simulink model "BLDC_motor"  (R2015b)
settings: Solver=VariableStepAuto  StartTime=0.0  StopTime=0.2  RelTol=1e-3
libraries: powerlib x15
settings Model: Creator=Meghdeep  LastModifiedBy=Jana

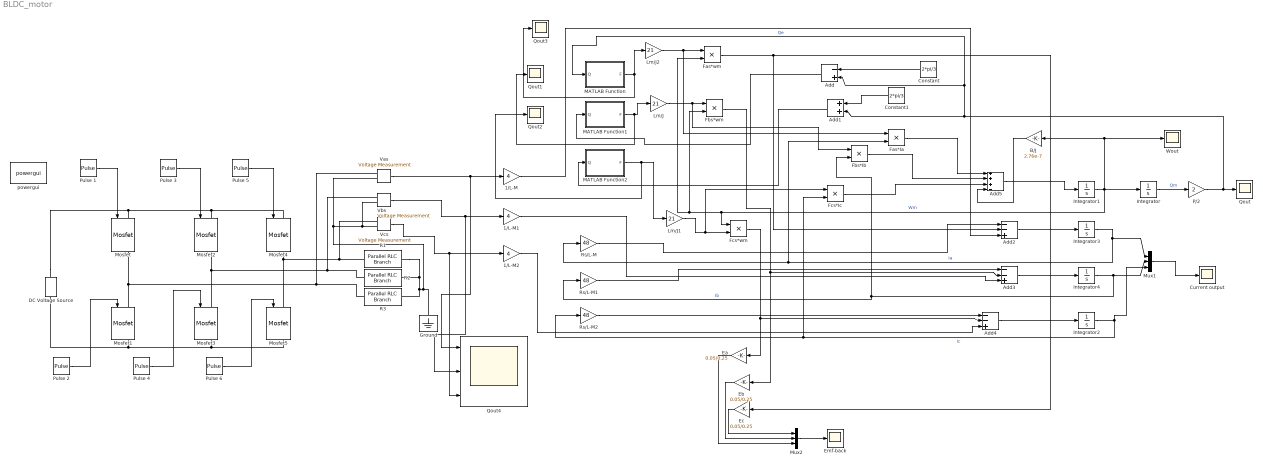
== system BLDC_motor ==
  1/L-M : Gain  Gain=4
  1/L-M1 : Gain  Gain=4
  1/L-M2 : Gain  Gain=4
  Add : Sum  Inputs=-+
  Add1 : Sum
  Add2 : Sum  Inputs=--+
  Add3 : Sum  Inputs=--+
  Add4 : Sum  Inputs=--+
  Add5 : Sum  Inputs=+++-
  B/J : Gain  Gain=2.76e-7
  Constant : Constant  Value=2*pi/3
  Constant1 : Constant  Value=2*pi/3
  Current output : Scope
  DC Voltage Source : powerlib/Electrical Sources/DC Voltage Source  Amplitude=10  Measurements=None
  Ea : Gain  Gain=0.05/0.25
  Eb : Gain  Gain=0.05/0.25
  Ec : Gain  Gain=0.05/0.25
  Emf-back : Scope
  Fas*Ia : Product
  Fas*wm : Product
  Fbs*Ib : Product
  Fbs*wm : Product
  Fcs*Ic : Product
  Fcs*wm : Product
  Ground : powerlib/Elements/Ground  LConnTagsString=a
  Integrator{,1..4} (5 alike) : Integrator
  Lm/J : Gain  Gain=21
  Lm/J1 : Gain  Gain=21
  Lm/J2 : Gain  Gain=21
  MATLAB Function : MATLAB Function  TreatAsAtomicUnit=on
  MATLAB Function1 : MATLAB Function  TreatAsAtomicUnit=on
  MATLAB Function2 : MATLAB Function  TreatAsAtomicUnit=on
  Mosfet{,1..5} (6 alike) : powerlib/Power Electronics/Mosfet  Ron=0.1  Lon=0  Rd=0.01  Vfd=0  IC=0  Rs=1e5  Cs=inf  Measurements=on
  Mux1 : Mux  Inputs=3
  Mux2 : Mux  Inputs=3
  P/2 : Gain  Gain=2
  Pulse 1 : DiscretePulseGenerator  PulseType=Time based  Amplitude=10  Period=0.02  PulseWidth=100/3
  Pulse 2 : DiscretePulseGenerator  PulseType=Time based  Amplitude=10  Period=0.02  PulseWidth=100/3  PhaseDelay=0.0033
  Pulse 3 : DiscretePulseGenerator  PulseType=Time based  Amplitude=10  Period=0.02  PulseWidth=100/3  PhaseDelay=0.0067
  Pulse 4 : DiscretePulseGenerator  PulseType=Time based  Amplitude=10  Period=0.02  PulseWidth=100/3  PhaseDelay=0.01
  Pulse 5 : DiscretePulseGenerator  PulseType=Time based  Amplitude=10  Period=0.02  PulseWidth=100/3  PhaseDelay=0.0133
  Pulse 6 : DiscretePulseGenerator  PulseType=Time based  Amplitude=10  Period=0.02  PulseWidth=100/3  PhaseDelay=0.0167
  Qout{,1..3} (4 alike) : Scope
  Qout4 : Scope  NumInputPorts=3
  R1 : powerlib/Elements/Parallel RLC Branch  LConnTagsString=a  RConnTagsString=__new0  BranchType=R  Resistance=1  Inductance=1e-3  SetiL0=off  InitialCurrent=0  Capacitance=1e-6  Setx0=off  InitialVoltage=0  Measurements=None
  R2 : powerlib/Elements/Parallel RLC Branch  LConnTagsString=a  RConnTagsString=__new0  BranchType=R  Resistance=1  Inductance=1e-3  SetiL0=off  InitialCurrent=0  Capacitance=1e-6  Setx0=off  InitialVoltage=0  Measurements=None
  R3 : powerlib/Elements/Parallel RLC Branch  LConnTagsString=a  RConnTagsString=__new0  BranchType=R  Resistance=1  Inductance=1e-3  SetiL0=off  InitialCurrent=0  Capacitance=1e-6  Setx0=off  InitialVoltage=0  Measurements=None
  Rs/L-M : Gain  Gain=48
  Rs/L-M1 : Gain  Gain=48
  Rs/L-M2 : Gain  Gain=48
  Vas : powerlib/Measurements/Voltage Measurement  PhasorSimulation=off  OutputType=Complex  PSBequivalent=0
  Vbs : powerlib/Measurements/Voltage Measurement  PhasorSimulation=off  OutputType=Complex  PSBequivalent=0
  Vcs : powerlib/Measurements/Voltage Measurement  PhasorSimulation=off  OutputType=Complex  PSBequivalent=0
  Wout : Scope
  powergui : powerlib/powergui  Priority=1  SimulationMode=Continuous  SolverType=Tustin/Backward Euler (TBE)  SampleTime=50e-6  frequency=60  SPID=off  DisableSnubberDevices=off  DisableRonSwitches=off  DisableVfSwitches=off  SwTol=0  DisplayEquations=off  Interpol=off  ExternalGateDelay=off  methode=off  Ts=10  FunctionMessages=off  echomessages=off  HookPort=off  EnableUseOfTLC=off  x0status=blocks  frequencyindice=0  Pbase=100e6  ErrMax=1e-4  Iterations=50  UnitsV=kV  UnitsW=MW  buscounter=0  RestoreLinks=warning  ResistiveCurrentMeasurement=off  Frange=[0:2:500]  Ylog=off  Xlog=on  ShowGrid=off  save=off  variable=ZData  structure=0  ZoomFFT=off  StartTime=0.0  cycles=1  DisplayStyle=1  fundamental=60  FreqAxis=off  MaxFrequency=1000  frequencyindicesteady=1  RmsSteady=1  display=off
  wires:
  Integrator1/1 -> B/J/1, Wout/1, Integrator/1, Fcs*wm/1, Fas*wm/2, Fbs*wm/2  "Wm"
  Integrator3/1 -> Mux1/1, Fas*Ia/2, Rs/L-M/1  "Ia"
  Integrator4/1 -> Mux1/2, Fbs*Ib/2, Rs/L-M1/1  "Ib"
  Integrator2/1 -> Mux1/3, Fcs*Ic/2, Rs/L-M2/1  "Ic"
  Fbs*wm/1 -> Add3/2, Eb/1
  P/2/1 -> Qout/1, MATLAB Function/1(Q), Add/2, Add1/2  "Qe"
  Constant/1 -> Add/1
  Constant1/1 -> Add1/1
  Add/1 -> MATLAB Function1/1(Q)
  Add1/1 -> MATLAB Function2/1(Q)
  Fcs*wm/1 -> Add4/2, Ea/1
  Fas*wm/1 -> Add2/2, Ec/1
  Lm/J2/1 -> Fas*wm/1, Fas*Ia/1
  1/L-M/1 -> Add2/3
  Rs/L-M/1 -> Add2/1
  Add2/1 -> Integrator3/1
  Rs/L-M1/1 -> Add3/1
  Lm/J/1 -> Fbs*Ib/1, Fbs*wm/1
  1/L-M1/1 -> Add3/3
  Rs/L-M2/1 -> Add4/1
  Lm/J1/1 -> Fcs*Ic/1, Fcs*wm/2
  1/L-M2/1 -> Add4/3
  Ec/1 -> Mux2/1
  Add3/1 -> Integrator4/1
  Add4/1 -> Integrator2/1
  B/J/1 -> Add5/4
  MATLAB Function1/1(F) -> Qout1/1, Lm/J/1
  MATLAB Function/1(F) -> Lm/J2/1, Qout3/1
  MATLAB Function2/1(F) -> Qout2/1, Lm/J1/1
  Fcs*Ic/1 -> Add5/3
  Fbs*Ib/1 -> Add5/2
  Fas*Ia/1 -> Add5/1
  Add5/1 -> Integrator1/1
  Mux1/1 -> Current output/1
  Eb/1 -> Mux2/2
  Ea/1 -> Mux2/3
  Mux2/1 -> Emf-back/1
  Pulse 5/1 -> Mosfet4/1
  Pulse 3/1 -> Mosfet2/1
  Pulse 1/1 -> Mosfet/1
  Pulse 6/1 -> Mosfet5/1
  Pulse 4/1 -> Mosfet3/1
  Pulse 2/1 -> Mosfet1/1
  Vas/1 -> Qout4/1, 1/L-M/1
  Vbs/1 -> Qout4/2, 1/L-M1/1
  Vcs/1 -> Qout4/3, 1/L-M2/1
  Integrator/1 -> P/2/1  "Qm"
  connections:
  DC Voltage Source/RConn1 -- Mosfet4/LConn1 -- Mosfet2/LConn1 -- Mosfet/LConn1
  Mosfet1/RConn1 -- Mosfet5/RConn1 -- Mosfet3/RConn1 -- DC Voltage Source/LConn1
  Mosfet/RConn1 -- Vas/LConn1 -- R3/LConn1 -- Mosfet1/LConn1
  Mosfet2/RConn1 -- Vbs/LConn1 -- R2/LConn1 -- Mosfet3/LConn1
  Mosfet4/RConn1 -- Vcs/LConn1 -- R1/LConn1 -- Mosfet5/LConn1
  R3/RConn1 -- Vas/LConn2 -- Vbs/LConn2 -- Vcs/LConn2 -- Ground/LConn1 -- R2/RConn1 -- R1/RConn1

== matlab function BLDC_motor/MATLAB Function1 ==
  data: Q input; F output
function F = trapez(Q)
%#codegen
Q = mod(Q,2*pi);
if Q >=0 && Q<2*pi/3
    F = 1;
elseif Q>= 2*pi/3 && Q< pi
    F = 1-6*(Q-2*pi/3)/pi;
elseif Q>= pi && Q<=5*pi/3
    F = -1;
elseif Q>= 5*pi/3 && Q<= 2*pi
    F = -1 + 6*(Q-5*pi/3)/pi;
end
F = Q;

== matlab function BLDC_motor/MATLAB Function ==
  data: Q input; F output
function F = trapez(Q)
%#codegen
Q = mod(Q,2*pi);
if Q >=0 && Q<2*pi/3
    F = 1;
elseif Q>= 2*pi/3 && Q< pi
    F = 1-6*(Q-2*pi/3)/pi;
elseif Q>= pi && Q<=5*pi/3
    F = -1;
elseif Q>= 5*pi/3 && Q<= 2*pi
    F = -1 + 6*(Q-5*pi/3)/pi;
end
F = Q;

== matlab function BLDC_motor/MATLAB Function2 ==
  data: Q input; F output
function F = trapez(Q)
%#codegen
Q = mod(Q,2*pi);
if Q >=0 && Q<2*pi/3
    F = 1;
elseif Q>= 2*pi/3 && Q< pi
    F = 1-6*(Q-2*pi/3)/pi;
elseif Q>= pi && Q<=5*pi/3
    F = -1;
elseif Q>= 5*pi/3 && Q<= 2*pi
    F = -1 + 6*(Q-5*pi/3)/pi;
end
F = Q;
